simulink model "chi2Test"  (R2020b)
settings: Solver=VariableStepAuto  StartTime=0.0  StopTime=10.0  RelTol=1e-3
values from neighbouring files (symbols this model uses):
  Ts = 0.1    [RLenv.m]    (also in RlEnvModel.m; envRL.mat; sys_env.m)
libraries: simulink x2
settings Model: EnablePacing=on  PacingRate=0.100000  Creator=IIT_KGP_CSE_FM_LAB  LastModifiedBy=IIT_KGP_CSE_FM_LAB

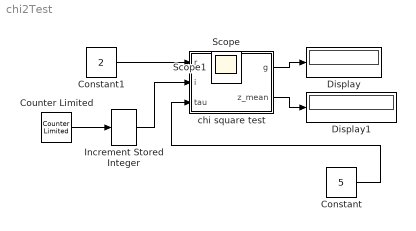
== system chi2Test ==
  Constant : Constant  Value=5  SampleTime=Ts
  Constant1 : Constant  Value=2  SampleTime=Ts
  Counter Limited : simulink/Sources/Counter Limited  uplimit=1/Ts-1  tsamp=Ts
  Display : Display
  Display1 : Display
  Increment Stored Integer : simulink/Additional Math & Discrete/Additional Math: Increment - Decrement/Increment Stored Integer
  chi square test : Subsystem
  Scope : Scope
  Scope1 : Scope
  wires:
  Counter Limited/1 -> Increment Stored Integer/1
  Constant/1 -> chi square test/3(tau)
  Constant1/1 -> chi square test/1(r)
  chi square test/1(g) -> Display/1
  chi square test/2(z_mean) -> Display1/1
  Increment Stored Integer/1 -> chi square test/2(i)

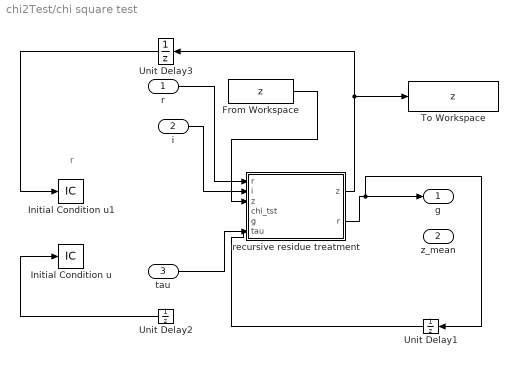
== system chi2Test/chi square test ==
  note: r
  r : Inport
  i : Inport  Port=2
  tau : Inport  Port=3
  From Workspace : FromWorkspace  VariableName=z  SampleTime=Ts
  Initial Condition u : InitialCondition  Value=[0]
  Initial Condition u1 : InitialCondition  Value=[0]
  To Workspace : ToWorkspace  VariableName=z  SampleTime=Ts
  Unit Delay1 : UnitDelay  SampleTime=Ts  HasFrameUpgradeWarning=on
  Unit Delay2 : UnitDelay  SampleTime=Ts  HasFrameUpgradeWarning=on
  Unit Delay3 : UnitDelay  InitialCondition=[0]  SampleTime=Ts  HasFrameUpgradeWarning=on
  recursive residue treatment : MATLAB Function  TreatAsAtomicUnit=on
  g : Outport
  z_mean : Outport  Port=2
  wires:
  Unit Delay2/1 -> Initial Condition u/1
  r/1 -> recursive residue treatment/1("r ")
  Unit Delay1/1 -> ?
  Unit Delay3/1 -> Initial Condition u1/1
  ? -> z_mean/1
  i/1 -> recursive residue treatment/2(i)
  ? -> Unit Delay2/1
  tau/1 -> recursive residue treatment/6(tau)
  recursive residue treatment/1(z) -> To Workspace/1, Unit Delay3/1
  recursive residue treatment/2(r) -> Unit Delay1/1, g/1
  From Workspace/1 -> recursive residue treatment/3("z ")

== matlab function chi2Test/chi square test/recursive residue treatment ==
  data: z output; r output; r input; i input; z input; chi_tst input; g input; tau input
function [z,r] = fcn(r,i,z,chi_tst,g,tau)
% function [g,z,z_mean,chi_tst] = fcn(r,i,z,chi_tst,g,tau)
z (:,i)= r;
% z_mean=mean(z)
% P= size(z',1)
% chi_tst(i)= z(:,i)'*z(:,i)/P
% g(i) = 0;              
% for k = max(1,i-tau+1):i
%     g(i) = g(i) + chi_tst(k)  % Calculate gk (chi2 test)
% end
